simulink model "Modelo_cinematico_2015"  (R2016a)
settings: Solver=FixedStepAuto  StartTime=0.0  StopTime=20.0  FixedStep=0.01  RelTol=1e-3
settings Model: Creator=daniel  LastModifiedBy=daniel
settings DataIOCC: ExternalInput=[b, d, r]  LimitDataPoints=on
settings DebuggingCC: AllowSymbolicDim=off
settings ModelReferenceCC: PropagateSignalLabelsOutOfModel=off
settings GRTTargetCC: GeneratePreprocessorConditionals=Use local settings

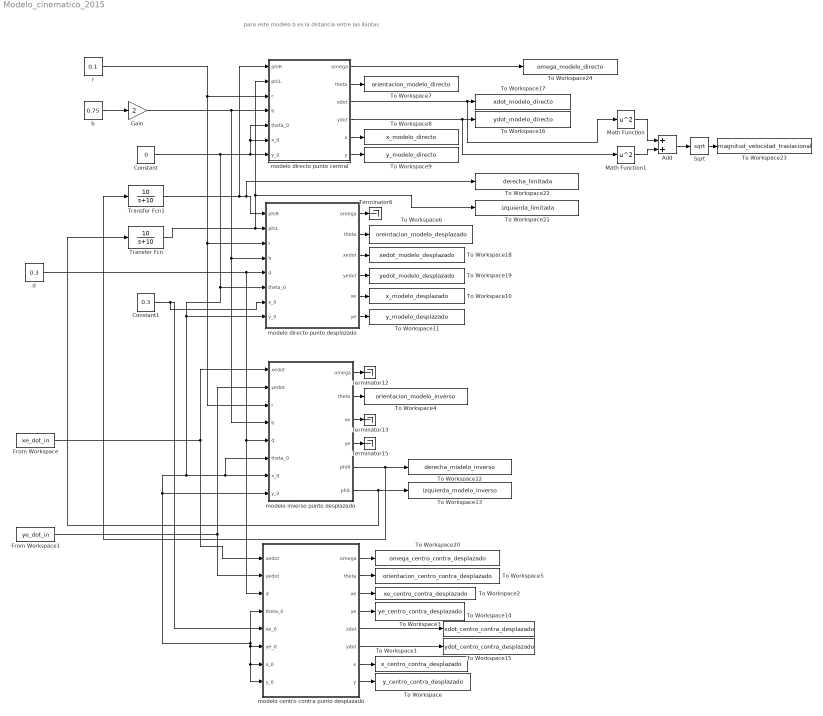
== system Modelo_cinematico_2015 ==
  note: para este modelo b es la distancia entre las llantas
  Add : Sum
  Constant : Constant  Value=0
  Constant1 : Constant  Value=0.3
  From Workspace : FromWorkspace  VariableName=xe_dot_in  SampleTime=0
  From Workspace1 : FromWorkspace  VariableName=ye_dot_in  SampleTime=0
  Gain : Gain  Gain=2
  Math Function : Math  Operator=square  SaturateOnIntegerOverflow=on
  Math Function1 : Math  Operator=square  SaturateOnIntegerOverflow=on
  Sqrt : Sqrt  SaturateOnIntegerOverflow=on
  Terminator{6,12..13,15} (4 alike) : Terminator
  To Workspace : ToWorkspace  VariableName=y_centro_contra_desplazado  SaveFormat=Timeseries  SampleTime=-1
  To Workspace1 : ToWorkspace  VariableName=x_centro_contra_desplazado  SaveFormat=Timeseries  SampleTime=-1
  To Workspace10 : ToWorkspace  VariableName=x_modelo_desplazado  SaveFormat=Timeseries  SampleTime=-1
  To Workspace11 : ToWorkspace  VariableName=y_modelo_desplazado  SaveFormat=Timeseries  SampleTime=-1
  To Workspace12 : ToWorkspace  VariableName=derecha_modelo_inverso  SaveFormat=Timeseries  SampleTime=-1
  To Workspace13 : ToWorkspace  VariableName=izquierda_modelo_inverso  SaveFormat=Timeseries  SampleTime=-1
  To Workspace14 : ToWorkspace  VariableName=xdot_centro_contra_desplazado  SaveFormat=Timeseries  SampleTime=-1
  To Workspace15 : ToWorkspace  VariableName=ydot_centro_contra_desplazado  SaveFormat=Timeseries  SampleTime=-1
  To Workspace16 : ToWorkspace  VariableName=ydot_modelo_directo  SaveFormat=Timeseries  SampleTime=-1
  To Workspace17 : ToWorkspace  VariableName=xdot_modelo_directo  SaveFormat=Timeseries  SampleTime=-1
  To Workspace18 : ToWorkspace  VariableName=xedot_modelo_desplazado  SaveFormat=Timeseries  SampleTime=-1
  To Workspace19 : ToWorkspace  VariableName=yedot_modelo_desplazado  SaveFormat=Timeseries  SampleTime=-1
  To Workspace2 : ToWorkspace  VariableName=xe_centro_contra_desplazado  SaveFormat=Timeseries  SampleTime=-1
  To Workspace20 : ToWorkspace  VariableName=omega_centro_contra_desplazado  SaveFormat=Timeseries  SampleTime=-1
  To Workspace21 : ToWorkspace  VariableName=izquierda_limitada  SaveFormat=Timeseries  SampleTime=-1
  To Workspace22 : ToWorkspace  VariableName=derecha_limitada  SaveFormat=Timeseries  SampleTime=-1
  To Workspace23 : ToWorkspace  VariableName=magnitud_velocidad_traslacional  SaveFormat=Timeseries  SampleTime=-1
  To Workspace24 : ToWorkspace  VariableName=omega_modelo_directo  SaveFormat=Timeseries  SampleTime=-1
  To Workspace3 : ToWorkspace  VariableName=ye_centro_contra_desplazado  SaveFormat=Timeseries  SampleTime=-1
  To Workspace4 : ToWorkspace  VariableName=orientacion_modelo_inverso  SaveFormat=Timeseries  SampleTime=-1
  To Workspace5 : ToWorkspace  VariableName=orientacion_centro_contra_desplazado  SaveFormat=Timeseries  SampleTime=-1
  To Workspace6 : ToWorkspace  VariableName=oreintacion_modelo_desplazado  SaveFormat=Timeseries  SampleTime=-1
  To Workspace7 : ToWorkspace  VariableName=orientacion_modelo_directo  SaveFormat=Timeseries  SampleTime=-1
  To Workspace8 : ToWorkspace  VariableName=x_modelo_directo  SaveFormat=Timeseries  SampleTime=-1
  To Workspace9 : ToWorkspace  VariableName=y_modelo_directo  SaveFormat=Timeseries  SampleTime=-1
  Transfer Fcn : TransferFcn  Numerator=[10]  Denominator=[1 10]
  Transfer Fcn1 : TransferFcn  Numerator=[10]  Denominator=[1 10]
  b : Constant  Value=0.75
  d : Constant  Value=0.3
  modelo centro contra punto desplazado : Subsystem
  modelo directo punto central : Subsystem
  modelo directo punto desplazado : Subsystem
  modelo inverso punto desplazado : Subsystem
  r : Constant  Value=0.1
  wires:
  modelo centro contra punto desplazado/8(y) -> To Workspace/1
  modelo centro contra punto desplazado/7(x) -> To Workspace1/1
  modelo centro contra punto desplazado/3(xe) -> To Workspace2/1
  modelo centro contra punto desplazado/4(ye) -> To Workspace3/1
  From Workspace1/1 -> modelo centro contra punto desplazado/2(yedot), modelo inverso punto desplazado/2(yedot)
  From Workspace/1 -> modelo inverso punto desplazado/1(xedot), modelo centro contra punto desplazado/1(xedot)
  Constant/1 -> modelo directo punto central/5(theta_0), modelo directo punto central/6(x_0), modelo directo punto central/7(y_0), modelo centro contra punto desplazado/8(y_0), modelo centro contra punto desplazado/7(x_0), modelo centro contra punto desplazado/6(ye_0), modelo centro contra punto desplazado/4(theta_0), modelo inverso punto desplazado/8(y_0), modelo inverso punto desplazado/6(theta_0), modelo inverso punto desplazado/7(x_0), modelo directo punto desplazado/8(y_0), modelo directo punto desplazado/6(theta_0)
  modelo directo punto central/3(xdot) -> Math Function/1, To Workspace17/1
  modelo directo punto central/4(ydot) -> Math Function1/1, To Workspace16/1
  modelo directo punto central/5(x) -> To Workspace8/1
  modelo directo punto central/6(y) -> To Workspace9/1
  modelo directo punto desplazado/1("omega ") -> Terminator6/1
  modelo directo punto desplazado/2(theta) -> To Workspace6/1
  modelo directo punto desplazado/3(xedot) -> To Workspace18/1
  modelo directo punto desplazado/4(yedot) -> To Workspace19/1
  modelo directo punto desplazado/5(xe) -> To Workspace10/1
  modelo directo punto desplazado/6(ye) -> To Workspace11/1
  modelo inverso punto desplazado/1("omega ") -> Terminator12/1
  modelo inverso punto desplazado/4(ye) -> Terminator15/1
  modelo centro contra punto desplazado/1("omega ") -> To Workspace20/1
  modelo centro contra punto desplazado/2(theta) -> To Workspace5/1
  modelo centro contra punto desplazado/5(xdot) -> To Workspace14/1
  modelo centro contra punto desplazado/6(ydot) -> To Workspace15/1
  modelo inverso punto desplazado/3(xe) -> Terminator13/1
  modelo inverso punto desplazado/2(theta) -> To Workspace4/1
  modelo directo punto central/1("omega ") -> To Workspace24/1
  modelo directo punto central/2(theta) -> To Workspace7/1
  Transfer Fcn/1 -> modelo directo punto central/2(phiL), To Workspace21/1, modelo directo punto desplazado/2(phiL)
  Transfer Fcn1/1 -> modelo directo punto central/1(phiR), To Workspace22/1, modelo directo punto desplazado/1(phiR)
  modelo inverso punto desplazado/5(phiR) -> Transfer Fcn1/1, To Workspace12/1
  modelo inverso punto desplazado/6(phiL) -> Transfer Fcn/1, To Workspace13/1
  Math Function/1 -> Add/1
  Math Function1/1 -> Add/2
  Add/1 -> Sqrt/1
  Sqrt/1 -> To Workspace23/1
  r/1 -> modelo inverso punto desplazado/3(r), modelo directo punto desplazado/3(r), modelo directo punto central/3(r)
  b/1 -> Gain/1
  d/1 -> modelo centro contra punto desplazado/3(d), modelo inverso punto desplazado/5(d), modelo directo punto desplazado/5(d)
  Constant1/1 -> modelo centro contra punto desplazado/5(xe_0), modelo directo punto desplazado/7(x_0)
  Gain/1 -> modelo inverso punto desplazado/4(b), modelo directo punto desplazado/4(b), modelo directo punto central/4(b)

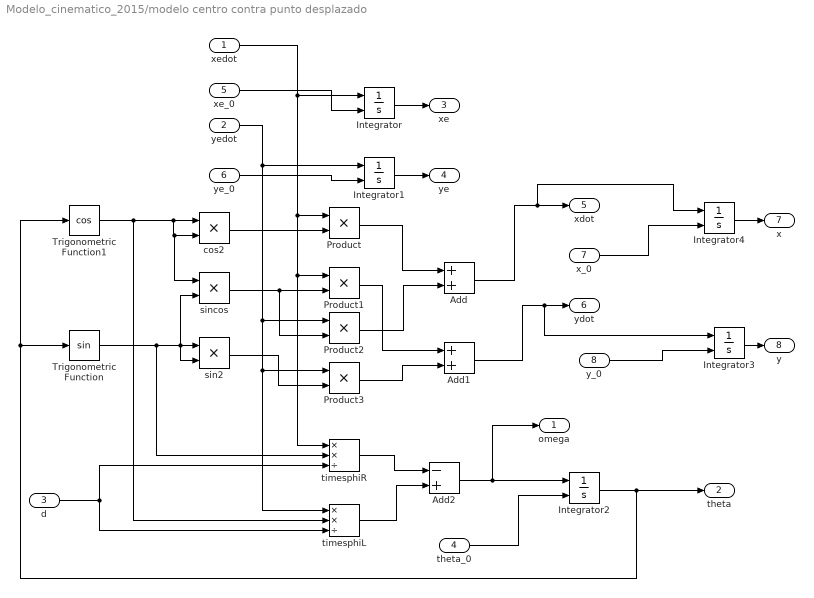
== system Modelo_cinematico_2015/modelo centro contra punto desplazado ==
  xedot : Inport
  yedot : Inport  Port=2
  d : Inport  Port=3
  theta_0 : Inport  Port=4
  xe_0 : Inport  Port=5
  ye_0 : Inport  Port=6
  x_0 : Inport  Port=7
  y_0 : Inport  Port=8
  Add : Sum
  Add1 : Sum
  Add2 : Sum  Inputs=-+
  Integrator{,1..4} (5 alike) : Integrator  InitialConditionSource=external
  Product{,1..3} (4 alike) : Product  Inputs=**
  Trigonometric Function : Trigonometry
  Trigonometric Function1 : Trigonometry  Operator=cos
  cos2 : Product  Inputs=**
  sin2 : Product  Inputs=**
  sincos : Product  Inputs=**
  timesphiL : Product  Inputs=**/
  timesphiR : Product  Inputs=**/
  "omega " : Outport
  theta : Outport  Port=2
  xe : Outport  Port=3
  ye : Outport  Port=4
  xdot : Outport  Port=5
  ydot : Outport  Port=6
  x : Outport  Port=7
  y : Outport  Port=8
  wires:
  Product1/1 -> Add1/1
  Add1/1 -> Integrator3/1, ydot/1
  yedot/1 -> Integrator1/1, timesphiL/1, Product3/1, Product2/1
  sincos/1 -> Product2/2, Product1/2
  d/1 -> timesphiR/3, timesphiL/3
  Trigonometric Function/1 -> timesphiR/2, sincos/2, sin2/2, sin2/1
  theta_0/1 -> Integrator2/2
  Integrator2/1 -> theta/1, Trigonometric Function1/1, Trigonometric Function/1
  xe_0/1 -> Integrator/2
  timesphiR/1 -> Add2/1
  Add/1 -> Integrator4/1, xdot/1
  Add2/1 -> "omega "/1, Integrator2/1
  cos2/1 -> Product/2
  xedot/1 -> Integrator/1, timesphiR/1, Product1/1, Product/1
  ye_0/1 -> Integrator1/2
  Product/1 -> Add/1
  Integrator/1 -> xe/1
  sin2/1 -> Product3/2
  Integrator1/1 -> ye/1
  Product2/1 -> Add/2
  Product3/1 -> Add1/2
  timesphiL/1 -> Add2/2
  Trigonometric Function1/1 -> timesphiL/2, sincos/1, cos2/2, cos2/1
  x_0/1 -> Integrator4/2
  y_0/1 -> Integrator3/2
  Integrator4/1 -> x/1
  Integrator3/1 -> y/1

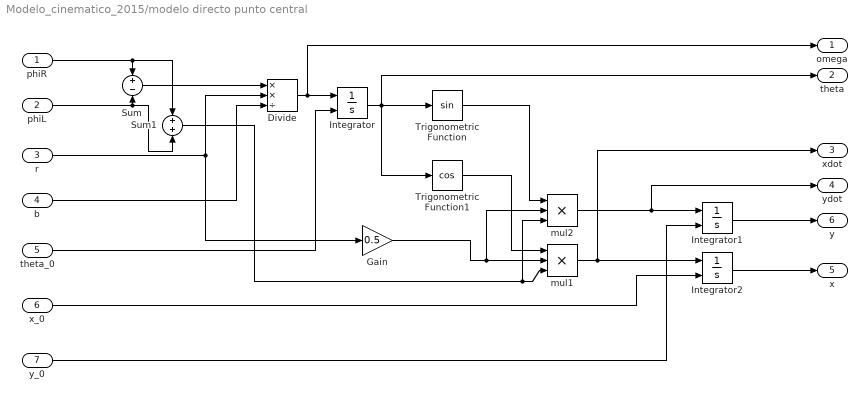
== system Modelo_cinematico_2015/modelo directo punto central ==
  phiR : Inport
  phiL : Inport  Port=2
  r : Inport  Port=3
  b : Inport  Port=4
  theta_0 : Inport  Port=5
  x_0 : Inport  Port=6
  y_0 : Inport  Port=7
  Divide : Product  Inputs=**/
  Gain : Gain  Gain=0.5
  Integrator : Integrator  InitialConditionSource=external
  Integrator1 : Integrator  InitialConditionSource=external
  Integrator2 : Integrator  InitialConditionSource=external
  Sum : Sum  Inputs=+-
  Sum1 : Sum
  Trigonometric Function : Trigonometry
  Trigonometric Function1 : Trigonometry  Operator=cos
  mul1 : Product  Inputs=***
  mul2 : Product  Inputs=***
  "omega " : Outport
  theta : Outport  Port=2
  xdot : Outport  Port=3
  ydot : Outport  Port=4
  x : Outport  Port=5
  y : Outport  Port=6
  wires:
  theta_0/1 -> Integrator/2
  Divide/1 -> "omega "/1, Integrator/1
  Sum/1 -> Divide/1
  r/1 -> Divide/2, Gain/1
  Sum1/1 -> mul2/3, mul1/3
  b/1 -> Divide/3
  phiL/1 -> Sum1/2, Sum/2
  Integrator/1 -> theta/1, Trigonometric Function1/1, Trigonometric Function/1
  Trigonometric Function1/1 -> mul1/1
  phiR/1 -> Sum1/1, Sum/1
  Integrator2/1 -> x/1
  Gain/1 -> mul2/2, mul1/2
  x_0/1 -> Integrator2/2
  mul2/1 -> ydot/1, Integrator1/1
  mul1/1 -> xdot/1, Integrator2/1
  Trigonometric Function/1 -> mul2/1
  Integrator1/1 -> y/1
  y_0/1 -> Integrator1/2

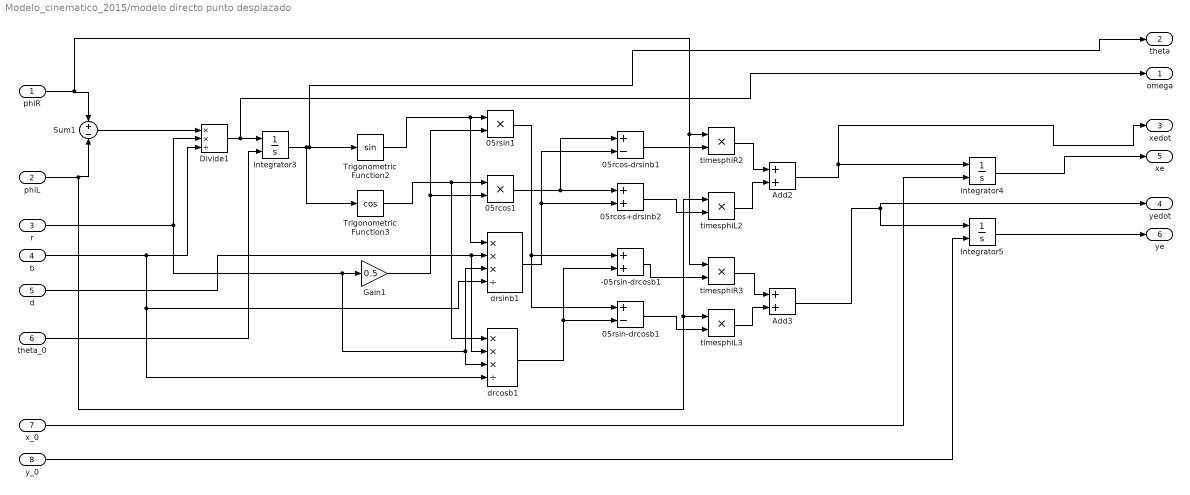
== system Modelo_cinematico_2015/modelo directo punto desplazado ==
  phiR : Inport
  phiL : Inport  Port=2
  r : Inport  Port=3
  b : Inport  Port=4
  d : Inport  Port=5
  theta_0 : Inport  Port=6
  x_0 : Inport  Port=7
  y_0 : Inport  Port=8
  -05rsin-drcosb1 : Sum
  05rcos+drsinb2 : Sum
  05rcos-drsinb1 : Sum  Inputs=+-
  05rcos1 : Product
  05rsin-drcosb1 : Sum  Inputs=+-
  05rsin1 : Product
  Add2 : Sum
  Add3 : Sum
  Divide1 : Product  Inputs=**/
  Gain1 : Gain  Gain=0.5
  Integrator3 : Integrator  InitialConditionSource=external
  Integrator4 : Integrator  InitialConditionSource=external
  Integrator5 : Integrator  InitialConditionSource=external
  Sum1 : Sum  Inputs=+-
  Trigonometric Function2 : Trigonometry
  Trigonometric Function3 : Trigonometry  Operator=cos
  drcosb1 : Product  Inputs=***/
  drsinb1 : Product  Inputs=***/
  timesphiL2 : Product  Inputs=**
  timesphiL3 : Product  Inputs=**
  timesphiR2 : Product  Inputs=**
  timesphiR3 : Product  Inputs=**
  "omega " : Outport
  theta : Outport  Port=2
  xedot : Outport  Port=3
  yedot : Outport  Port=4
  xe : Outport  Port=5
  ye : Outport  Port=6
  wires:
  Add3/1 -> yedot/1, Integrator5/1
  y_0/1 -> Integrator5/2
  b/1 -> drcosb1/4, drsinb1/4, Divide1/3
  timesphiR2/1 -> Add2/1
  05rsin1/1 -> 05rsin-drcosb1/1, -05rsin-drcosb1/1
  drcosb1/1 -> 05rsin-drcosb1/2, -05rsin-drcosb1/2
  drsinb1/1 -> 05rcos+drsinb2/2, 05rcos-drsinb1/2
  Trigonometric Function3/1 -> drcosb1/1, 05rcos1/1
  Gain1/1 -> 05rsin1/2, 05rcos1/2
  Integrator5/1 -> ye/1
  timesphiR3/1 -> Add3/1
  Divide1/1 -> "omega "/1, Integrator3/1
  05rcos-drsinb1/1 -> timesphiR2/2
  timesphiL2/1 -> Add2/2
  theta_0/1 -> Integrator3/2
  x_0/1 -> Integrator4/2
  d/1 -> drcosb1/2, drsinb1/2
  Sum1/1 -> Divide1/1
  05rcos+drsinb2/1 -> timesphiL2/2
  Trigonometric Function2/1 -> drsinb1/1, 05rsin1/1
  05rcos1/1 -> 05rcos+drsinb2/1, 05rcos-drsinb1/1
  phiR/1 -> Sum1/1, timesphiR3/1, timesphiR2/1
  Add2/1 -> xedot/1, Integrator4/1
  Integrator4/1 -> xe/1
  r/1 -> Divide1/2, drsinb1/3, drcosb1/3, Gain1/1
  Integrator3/1 -> Trigonometric Function3/1, theta/1, Trigonometric Function2/1
  phiL/1 -> Sum1/2, timesphiL3/1, timesphiL2/1
  05rsin-drcosb1/1 -> timesphiL3/2
  timesphiL3/1 -> Add3/2
  -05rsin-drcosb1/1 -> timesphiR3/2

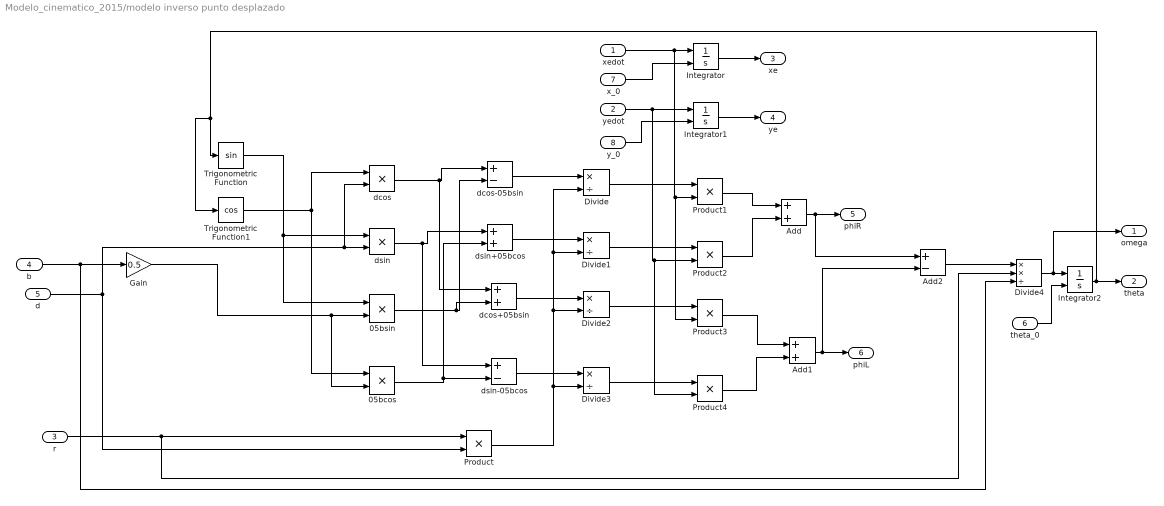
== system Modelo_cinematico_2015/modelo inverso punto desplazado ==
  xedot : Inport
  yedot : Inport  Port=2
  r : Inport  Port=3
  b : Inport  Port=4
  d : Inport  Port=5
  theta_0 : Inport  Port=6
  x_0 : Inport  Port=7
  y_0 : Inport  Port=8
  05bcos : Product  Inputs=**
  05bsin : Product  Inputs=**
  Add : Sum
  Add1 : Sum
  Add2 : Sum  Inputs=+-
  Divide{,1..3} (4 alike) : Product  Inputs=*/
  Divide4 : Product  Inputs=**/
  Gain : Gain  Gain=0.5
  Integrator : Integrator  InitialConditionSource=external
  Integrator1 : Integrator  InitialConditionSource=external
  Integrator2 : Integrator  InitialConditionSource=external
  Product{,1..4} (5 alike) : Product  Inputs=**
  Trigonometric Function : Trigonometry
  Trigonometric Function1 : Trigonometry  Operator=cos
  dcos : Product  Inputs=**
  dcos+05bsin : Sum
  dcos-05bsin : Sum  Inputs=+-
  dsin : Product  Inputs=**
  dsin+05bcos : Sum
  dsin-05bcos : Sum  Inputs=+-
  "omega " : Outport
  theta : Outport  Port=2
  xe : Outport  Port=3
  ye : Outport  Port=4
  phiR : Outport  Port=5
  phiL : Outport  Port=6
  wires:
  Product4/1 -> Add1/2
  yedot/1 -> Integrator1/1, Product4/2, Product2/2
  Integrator/1 -> xe/1
  theta_0/1 -> Integrator2/2
  Product3/1 -> Add1/1
  Product1/1 -> Add/1
  Integrator2/1 -> theta/1, Trigonometric Function1/1, Trigonometric Function/1
  Product2/1 -> Add/2
  Trigonometric Function/1 -> 05bsin/1, dsin/1
  Add1/1 -> phiL/1, Add2/2
  dsin/1 -> dsin-05bcos/1, dsin+05bcos/1
  y_0/1 -> Integrator1/2
  Divide4/1 -> "omega "/1, Integrator2/1
  xedot/1 -> Integrator/1, Product3/2, Product1/2
  r/1 -> Divide4/2, Product/1
  dsin+05bcos/1 -> Divide1/1
  Gain/1 -> 05bcos/2, 05bsin/2
  d/1 -> Product/2, dcos/2, dsin/2
  05bsin/1 -> dcos+05bsin/2, dcos-05bsin/2
  Add/1 -> phiR/1, Add2/1
  Add2/1 -> Divide4/1
  05bcos/1 -> dsin-05bcos/2, dsin+05bcos/2
  dcos/1 -> dcos+05bsin/1, dcos-05bsin/1
  Integrator1/1 -> ye/1
  x_0/1 -> Integrator/2
  Product/1 -> Divide/2, Divide1/2, Divide2/2, Divide3/2
  Trigonometric Function1/1 -> dcos/1, 05bcos/1
  Divide/1 -> Product1/1
  Divide2/1 -> Product3/1
  Divide3/1 -> Product4/1
  dcos-05bsin/1 -> Divide/1
  dcos+05bsin/1 -> Divide2/1
  Divide1/1 -> Product2/1
  dsin-05bcos/1 -> Divide3/1
  b/1 -> Divide4/3, Gain/1
